simulink model "Robot"  (R2018a)
settings: Solver=VariableStepAuto  StartTime=0.0  StopTime=inf  FixedStep=1e-4  RelTol=1e-3  EnableMultiTasking=on
values from neighbouring files (symbols this model uses):
  CM730_acc_center = (4 * 9.80665)    (= 39.2266)    [CM730.m]
  CM730_acc_gain = 512 / CM730_acc_center    (= 13.0523675261)    [CM730.m]
  CM730_gyro_center = (1600 / 360 * 2 * pi)    (= 27.9252680319)    [CM730.m]
  CM730_gyro_gain = 512 / CM730_gyro_center    (= 18.3346494442)    [CM730.m]
  CM730_sample_time = 1e-3    (= 0.001)    [CM730.m]
  FSR_max = 254    [FSR.m]
  FSR_no_load = 255    [FSR.m]
  FSR_sample_time = 0.001    [FSR.m]
  FSR_scale = 1000    [FSR.m]
  g = 0    [Euler.m]
  MX106_Te = 1/1000    (= 0.001)    [MX106_init.m]
  MX28_inertia = 9e-8 * MX28_reduction^2    (= 0.0033385284)    [MX28_init.m]
  MX28_Te = 1/1000    (= 0.001)    [MX28_init.m]
  posZero_ID1 = posZero(1)    [Robot_init.m]
  posZero_ID10 = posZero(14)    [Robot_init.m]
  posZero_ID11 = posZero(9)    [Robot_init.m]
  posZero_ID12 = posZero(15)    [Robot_init.m]
  posZero_ID13 = posZero(10)    [Robot_init.m]
  posZero_ID14 = posZero(16)    [Robot_init.m]
  posZero_ID15 = posZero(11)    [Robot_init.m]
  posZero_ID16 = posZero(17)    [Robot_init.m]
  posZero_ID17 = posZero(12)    [Robot_init.m]
  posZero_ID18 = posZero(18)    [Robot_init.m]
  posZero_ID19 = posZero(19)    [Robot_init.m]
  posZero_ID2 = posZero(4)    [Robot_init.m]
  posZero_ID20 = posZero(20)    [Robot_init.m]
  posZero_ID3 = posZero(2)    [Robot_init.m]
  posZero_ID4 = posZero(5)    [Robot_init.m]
  posZero_ID5 = posZero(3)    [Robot_init.m]
  posZero_ID6 = posZero(6)    [Robot_init.m]
  posZero_ID7 = posZero(7)    [Robot_init.m]
  posZero_ID8 = posZero(13)    [Robot_init.m]
  posZero_ID9 = posZero(8)    [Robot_init.m]
  robot_chest_mass = 2385.0    (= 2385)    [Robot_init.m]
  robot_floor_friction_coeff = 0.6    [Robot_init.m]
  robot_floor_position_gain = -1e5    (= -100000)    [Robot_init.m]
  robot_floor_speed_gain = -1e3    (= -1000)    [Robot_init.m]
  robot_gravity = [0 0 0]    [Robot_init.m]
  robot_head_mass = 177.69    [Robot_init.m]
  robot_hip1_mass = 49.00    (= 49)    [Robot_init.m]
  robot_left_ankle_mass = 360.00    (= 360)    [Robot_init.m]
  robot_left_foot_mass = 267.00    (= 267)    [Robot_init.m]
  robot_left_forearm_mass = 248.00    (= 248)    [Robot_init.m]
  robot_left_hip2_mass = 358.00    (= 358)    [Robot_init.m]
  robot_left_lower_leg_mass = 129.00    (= 129)    [Robot_init.m]
  robot_left_shoulder_mass = 39.00    (= 39)    [Robot_init.m]
  robot_left_thigh_mass = 1263.00    (= 1263)    [Robot_init.m]
  robot_left_upper_arm_mass = 247.00    (= 247)    [Robot_init.m]
  robot_neck_mass = 90    [Robot_init.m]
  robot_right_ankle_mass = 360.00    (= 360)    [Robot_init.m]
  robot_right_foot_mass = 267.00    (= 267)    [Robot_init.m]
  robot_right_forearm_mass = 248.00    (= 248)    [Robot_init.m]
  robot_right_hip2_mass = 358.00    (= 358)    [Robot_init.m]
  robot_right_lower_leg_mass = 129.00    (= 129)    [Robot_init.m]
  robot_right_shoulder_mass = 39.00    (= 39)    [Robot_init.m]
  robot_right_thigh_mass = 263.00    (= 263)    [Robot_init.m]
  robot_right_upper_arm_mass = 247.00    (= 247)    [Robot_init.m]
  X = get(hObject,'Value')    [gui_kine.m]
  Y = get(hObject,'Value')    [gui_kine.m]
  Z = get(hObject,'Value')    [gui_kine.m]
libraries: sm_lib x167, fl_lib x128, nesl_utility x77, dspindex x1
(part 2 of 7)

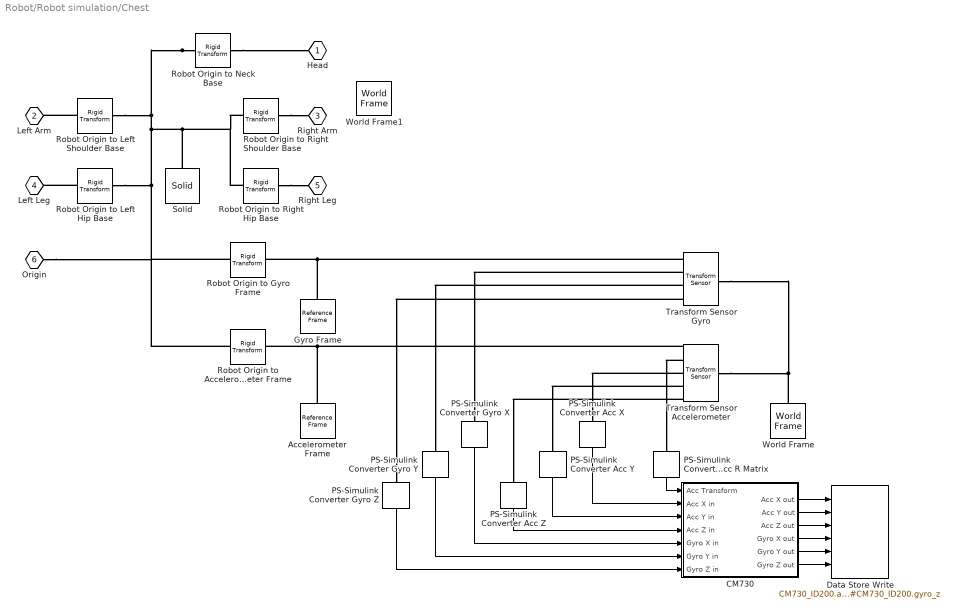
== system Robot/Robot simulation/Chest ==
  Accelerometer Frame : sm_lib/Frames and Transforms/Reference Frame
  CM730 : Subsystem  TreatAsAtomicUnit=on  SystemSampleTime=CM730_sample_time
  Data Store Write : DataStoreWrite  DataStoreName=CM730_ID200  DataStoreElements=CM730_ID200.acc_x#CM730_ID200.acc_y#CM730_ID200.acc_z#CM730_ID200.gyro_x#CM730_ID200.gyro_y#CM730_ID200.gyro_z
  Gyro Frame : sm_lib/Frames and Transforms/Reference Frame
  PS-Simulink Converter Acc R Matrix : nesl_utility/PS-Simulink Converter  PhysicalDomain=network_engine_domain  SubClassName=ps_output  LeftPortType=input  RightPortType=output  PseudoPeriodic=off  Frequencies=[]  Unit=1  AffineConversion=off
  PS-Simulink Converter Acc X : nesl_utility/PS-Simulink Converter  PhysicalDomain=network_engine_domain  SubClassName=ps_output  LeftPortType=input  RightPortType=output  PseudoPeriodic=off  Frequencies=[]  Unit=m/s^2  AffineConversion=off
  PS-Simulink Converter Acc Y : nesl_utility/PS-Simulink Converter  PhysicalDomain=network_engine_domain  SubClassName=ps_output  LeftPortType=input  RightPortType=output  PseudoPeriodic=off  Frequencies=[]  Unit=m/s^2  AffineConversion=off
  PS-Simulink Converter Acc Z : nesl_utility/PS-Simulink Converter  PhysicalDomain=network_engine_domain  SubClassName=ps_output  LeftPortType=input  RightPortType=output  PseudoPeriodic=off  Frequencies=[]  Unit=m/s^2  AffineConversion=off
  PS-Simulink Converter Gyro X : nesl_utility/PS-Simulink Converter  PhysicalDomain=network_engine_domain  SubClassName=ps_output  LeftPortType=input  RightPortType=output  PseudoPeriodic=off  Frequencies=[]  Unit=rad/s  AffineConversion=off
  PS-Simulink Converter Gyro Y : nesl_utility/PS-Simulink Converter  PhysicalDomain=network_engine_domain  SubClassName=ps_output  LeftPortType=input  RightPortType=output  PseudoPeriodic=off  Frequencies=[]  Unit=rad/s  AffineConversion=off
  PS-Simulink Converter Gyro Z : nesl_utility/PS-Simulink Converter  PhysicalDomain=network_engine_domain  SubClassName=ps_output  LeftPortType=input  RightPortType=output  PseudoPeriodic=off  Frequencies=[]  Unit=rad/s  AffineConversion=off
  Robot Origin to Accelerometer Frame : sm_lib/Frames and Transforms/Rigid Transform  TranslationMethod=Cartesian  TranslationStandardOffset=0  TranslationLengthUnit=mm  TranslationStandardAxis=+Z  TranslationCartesianOffset=robot_origin_to_acc_tra  TranslationROffset=0  TranslationROffsetUnits=m  TranslationZOffset=0  TranslationZOffsetUnits=m  TranslationThetaOffset=0  TranslationThetaOffsetUnits=deg  RotationMethod=RotationMatrix  RotationAngleUnits=deg  RotationStandardAxis=+Z  RotationAngle=0  RotationArbitraryAxis=[0 0 1]  FollAlignAxisA=+X  BaseAlignAxisA=-Y  FollAlignAxisB=+Z  BaseAlignAxisB=+Z  RotationSequenceAxes=FollowerAxes  RotationSequence=XYX  RotationSequenceAngles=[0 0 0]  RotationSequenceAnglesUnits=deg  RotationMatrix=robot_origin_to_acc_rot
  Robot Origin to Gyro Frame : sm_lib/Frames and Transforms/Rigid Transform  TranslationMethod=Cartesian  TranslationStandardOffset=0  TranslationLengthUnit=mm  TranslationStandardAxis=+Z  TranslationCartesianOffset=robot_origin_to_gyro_tra  TranslationROffset=0  TranslationROffsetUnits=m  TranslationZOffset=0  TranslationZOffsetUnits=m  TranslationThetaOffset=0  TranslationThetaOffsetUnits=deg  RotationMethod=RotationMatrix  RotationAngleUnits=deg  RotationStandardAxis=+Z  RotationAngle=0  RotationArbitraryAxis=[0 0 1]  FollAlignAxisA=+X  BaseAlignAxisA=-Y  FollAlignAxisB=+Z  BaseAlignAxisB=-Z  RotationSequenceAxes=FollowerAxes  RotationSequence=XYX  RotationSequenceAngles=[0 0 0]  RotationSequenceAnglesUnits=deg  RotationMatrix=robot_origin_to_gyro_rot
  Robot Origin to Left Hip Base : sm_lib/Frames and Transforms/Rigid Transform  TranslationMethod=Cartesian  TranslationStandardOffset=0  TranslationLengthUnit=mm  TranslationStandardAxis=+Z  TranslationCartesianOffset=robot_origin_to_left_hip_base_tra  TranslationROffset=0  TranslationROffsetUnits=m  TranslationZOffset=0  TranslationZOffsetUnits=m  TranslationThetaOffset=0  TranslationThetaOffsetUnits=deg  RotationMethod=RotationMatrix  RotationAngleUnits=deg  RotationStandardAxis=+Z  RotationAngle=0  RotationArbitraryAxis=[0 0 1]  FollAlignAxisA=+X  BaseAlignAxisA=-Y  FollAlignAxisB=+Y  BaseAlignAxisB=-X  RotationSequenceAxes=FollowerAxes  RotationSequence=XYX  RotationSequenceAngles=[0 0 0]  RotationSequenceAnglesUnits=deg  RotationMatrix=robot_origin_to_left_hip_base_rot
  Robot Origin to Left Shoulder Base : sm_lib/Frames and Transforms/Rigid Transform  TranslationMethod=Cartesian  TranslationStandardOffset=0  TranslationLengthUnit=mm  TranslationStandardAxis=+Z  TranslationCartesianOffset=robot_origin_to_left_shoulder_base_tra  TranslationROffset=0  TranslationROffsetUnits=m  TranslationZOffset=0  TranslationZOffsetUnits=m  TranslationThetaOffset=0  TranslationThetaOffsetUnits=deg  RotationMethod=RotationMatrix  RotationAngleUnits=deg  RotationStandardAxis=+Z  RotationAngle=0  RotationArbitraryAxis=[0 0 1]  FollAlignAxisA=+X  BaseAlignAxisA=+Y  FollAlignAxisB=+Y  BaseAlignAxisB=+Z  RotationSequenceAxes=FollowerAxes  RotationSequence=XYX  RotationSequenceAngles=[0 0 0]  RotationSequenceAnglesUnits=deg  RotationMatrix=robot_origin_to_left_shoulder_base_rot
  Robot Origin to Neck Base : sm_lib/Frames and Transforms/Rigid Transform  TranslationMethod=Cartesian  TranslationStandardOffset=0  TranslationLengthUnit=mm  TranslationStandardAxis=+Z  TranslationCartesianOffset=robot_origin_to_neck_base_tra  TranslationROffset=0  TranslationROffsetUnits=m  TranslationZOffset=0  TranslationZOffsetUnits=m  TranslationThetaOffset=0  TranslationThetaOffsetUnits=deg  RotationMethod=RotationMatrix  RotationAngleUnits=deg  RotationStandardAxis=+Z  RotationAngle=0  RotationArbitraryAxis=[0 0 1]  FollAlignAxisA=+X  BaseAlignAxisA=+Y  FollAlignAxisB=+Y  BaseAlignAxisB=+Z  RotationSequenceAxes=FollowerAxes  RotationSequence=XYX  RotationSequenceAngles=[0 0 0]  RotationSequenceAnglesUnits=deg  RotationMatrix=robot_origin_to_neck_base_rot
  Robot Origin to Right Hip Base : sm_lib/Frames and Transforms/Rigid Transform  TranslationMethod=Cartesian  TranslationStandardOffset=0  TranslationLengthUnit=mm  TranslationStandardAxis=+Z  TranslationCartesianOffset=robot_origin_to_right_hip_base_tra  TranslationROffset=0  TranslationROffsetUnits=m  TranslationZOffset=0  TranslationZOffsetUnits=m  TranslationThetaOffset=0  TranslationThetaOffsetUnits=deg  RotationMethod=RotationMatrix  RotationAngleUnits=deg  RotationStandardAxis=+Z  RotationAngle=0  RotationArbitraryAxis=[0 0 1]  FollAlignAxisA=+X  BaseAlignAxisA=-Y  FollAlignAxisB=+Y  BaseAlignAxisB=-X  RotationSequenceAxes=FollowerAxes  RotationSequence=XYX  RotationSequenceAngles=[0 0 0]  RotationSequenceAnglesUnits=deg  RotationMatrix=robot_origin_to_right_hip_base_rot
  Robot Origin to Right Shoulder Base : sm_lib/Frames and Transforms/Rigid Transform  TranslationMethod=Cartesian  TranslationStandardOffset=0  TranslationLengthUnit=mm  TranslationStandardAxis=+Z  TranslationCartesianOffset=robot_origin_to_right_shoulder_base_tra  TranslationROffset=0  TranslationROffsetUnits=m  TranslationZOffset=0  TranslationZOffsetUnits=m  TranslationThetaOffset=0  TranslationThetaOffsetUnits=deg  RotationMethod=RotationMatrix  RotationAngleUnits=deg  RotationStandardAxis=+Z  RotationAngle=0  RotationArbitraryAxis=[0 0 1]  FollAlignAxisA=-Z  BaseAlignAxisA=+X  FollAlignAxisB=-X  BaseAlignAxisB=+Y  RotationSequenceAxes=FollowerAxes  RotationSequence=XYX  RotationSequenceAngles=[0 0 0]  RotationSequenceAnglesUnits=deg  RotationMatrix=robot_origin_to_right_shoulder_base_rot
  Solid : sm_lib/Body Elements/Solid  InertiaType=Custom  Mass=robot_chest_mass  MassUnits=g  CenterOfMass=robot_origin_to_center_mass  CenterOfMassUnits=mm  MomentsOfInertia=robot_chest_moment_inertia  MomentsOfInertiaUnits=g*mm^2  ProductsOfInertia=robot_chest_product_inertia  ProductsOfInertiaUnits=g*mm^2  DensityBased=on  Density=1000  DensityUnits=kg/(m^3)  DoExposeReferenceFrame=on  SerializedFrames=<Frames/>  GraphicType=FromGeometry  MarkerShape=Sphere  MarkerSize=10  MarkerSizeUnits=m  GraphicVisPropType=SimpleVisualProperties  GraphicDiffuseColor=[0.5 0.5 0.5]  GraphicSpecularColor=[0.5 0.5 0.5 1.0]  GraphicAmbientColor=[0.15 0.15 0.15 1.0]  GraphicEmissiveColor=[0.0 0.0 0.0 1.0]  GraphicShininess=75  GraphicOpacity=1.0  GeometryShape=FromFile  RectangleSize=[1 1]  RectangleSizeUnits=m  BrickDimensions=[115.5 112.1 47.8]  BrickDimensionUnits=mm  CylinderRadius=1  CylinderRadiusUnits=m  CylinderLength=1  CylinderLengthUnits=m  SphereRadius=1  SphereRadiusUnits=m  EllipsoidRadii=[1 1 1]  EllipsoidRadiiUnits=m  ExtrusionCrossSection=[1 1; -1 1; -1 -1; 1 -1]  ExtrusionCrossSectionUnits=m  ExtrusionLength=1  ExtrusionLengthUnits=m  PolygonNumSides=3  PolygonOuterRadius=1  PolygonOuterRadiusUnits=m  ExtGeomFileType=STL  ExtGeomFileName=\STL\Chest.STL  ExtGeomFileUnits=mm  RevolutionCrossSection=[1 1; 1 -1; 2 -1; 2 1]  RevolutionCrossSectionUnits=m  RevolutionExtent=Full  RevolutionAngle=180  RevolutionAngleUnits=deg
  Transform Sensor Accelerometer : sm_lib/Frames and Transforms/Transform Sensor  MeasurementFrame=Follower  SenseAngle=off  SenseAxis=off  SenseAngle1=off  SenseAngle2=off  SenseAngle3=off  SenseQ=off  SenseR=on  SenseOmegaX=off  SenseOmegaY=off  SenseOmegaZ=off  SenseOmega1=off  SenseOmega2=off  SenseOmega3=off  SenseQDot=off  SenseRDot=off  SenseAlphaX=off  SenseAlphaY=off  SenseAlphaZ=off  SenseAlpha1=off  SenseAlpha2=off  SenseAlpha3=off  SenseQDDot=off  SenseRDDot=off  SenseX=off  SenseY=off  SenseZ=off  SenseRad=off  SenseAzim=off  SenseDist=off  SenseInc=off  SenseXDot=off  SenseYDot=off  SenseZDot=off  SenseRadDot=off  SenseAzimDot=off  SenseDistDot=off  SenseIncDot=off  SenseXDDot=on  SenseYDDot=on  SenseZDDot=on  SenseRadDDot=off  SenseAzimDDot=off  SenseDistDDot=off  SenseIncDDot=off
  Transform Sensor Gyro : sm_lib/Frames and Transforms/Transform Sensor  MeasurementFrame=Follower  SenseAngle=off  SenseAxis=off  SenseAngle1=off  SenseAngle2=off  SenseAngle3=off  SenseQ=off  SenseR=off  SenseOmegaX=on  SenseOmegaY=on  SenseOmegaZ=on  SenseOmega1=off  SenseOmega2=off  SenseOmega3=off  SenseQDot=off  SenseRDot=off  SenseAlphaX=off  SenseAlphaY=off  SenseAlphaZ=off  SenseAlpha1=off  SenseAlpha2=off  SenseAlpha3=off  SenseQDDot=off  SenseRDDot=off  SenseX=off  SenseY=off  SenseZ=off  SenseRad=off  SenseAzim=off  SenseDist=off  SenseInc=off  SenseXDot=off  SenseYDot=off  SenseZDot=off  SenseRadDot=off  SenseAzimDot=off  SenseDistDot=off  SenseIncDot=off  SenseXDDot=off  SenseYDDot=off  SenseZDDot=off  SenseRadDDot=off  SenseAzimDDot=off  SenseDistDDot=off  SenseIncDDot=off
  World Frame : sm_lib/Frames and Transforms/World Frame
  World Frame1 : sm_lib/Frames and Transforms/World Frame
  Head : PMIOPort  Side=Right
  Left Arm : PMIOPort  Port=2  Side=Left
  Right Arm : PMIOPort  Port=3  Side=Right
  Left Leg : PMIOPort  Port=4  Side=Left
  Right Leg : PMIOPort  Port=5  Side=Right
  Origin : PMIOPort  Port=6  Side=Left
  wires:
  CM730/1(Acc X out) -> Data Store Write/1
  CM730/2(Acc Y out) -> Data Store Write/2
  CM730/3(Acc Z out) -> Data Store Write/3
  CM730/4(Gyro X out) -> Data Store Write/4
  CM730/5(Gyro Y out) -> Data Store Write/5
  CM730/6(Gyro Z out) -> Data Store Write/6
  PS-Simulink Converter Acc X/1 -> CM730/2(Acc X in)
  PS-Simulink Converter Acc Y/1 -> CM730/3(Acc Y in)
  PS-Simulink Converter Acc Z/1 -> CM730/4(Acc Z in)
  PS-Simulink Converter Gyro X/1 -> CM730/5(Gyro X in)
  PS-Simulink Converter Gyro Z/1 -> CM730/7(Gyro Z in)
  PS-Simulink Converter Gyro Y/1 -> CM730/6(Gyro Y in)
  PS-Simulink Converter Acc R Matrix/1 -> CM730/1(Acc Transform)
  connections:
  Robot Origin to Neck Base/RConn1 -- Head/RConn1
  Robot Origin to Right Shoulder Base/RConn1 -- Right Arm/RConn1
  Robot Origin to Right Hip Base/RConn1 -- Right Leg/RConn1
  Robot Origin to Neck Base/LConn1 -- Robot Origin to Left Shoulder Base/LConn1 -- Robot Origin to Accelerometer Frame/LConn1 -- Origin/RConn1 -- Robot Origin to Gyro Frame/LConn1 -- Robot Origin to Left Hip Base/LConn1 -- Robot Origin to Right Hip Base/LConn1 -- Robot Origin to Right Shoulder Base/LConn1 -- Solid/RConn1
  Robot Origin to Left Shoulder Base/RConn1 -- Left Arm/RConn1
  Robot Origin to Left Hip Base/RConn1 -- Left Leg/RConn1
  Gyro Frame/RConn1 -- Transform Sensor Gyro/RConn1 -- Robot Origin to Gyro Frame/RConn1
  Accelerometer Frame/RConn1 -- Transform Sensor Accelerometer/RConn1 -- Robot Origin to Accelerometer Frame/RConn1
  World Frame/RConn1 -- Transform Sensor Gyro/LConn1 -- Transform Sensor Accelerometer/LConn1
  Transform Sensor Gyro/RConn2 -- PS-Simulink Converter Gyro X/LConn1
  Transform Sensor Gyro/RConn3 -- PS-Simulink Converter Gyro Y/LConn1
  Transform Sensor Gyro/RConn4 -- PS-Simulink Converter Gyro Z/LConn1
  Transform Sensor Accelerometer/RConn2 -- PS-Simulink Converter Acc R Matrix/LConn1
  Transform Sensor Accelerometer/RConn5 -- PS-Simulink Converter Acc Z/LConn1
  Transform Sensor Accelerometer/RConn4 -- PS-Simulink Converter Acc Y/LConn1
  Transform Sensor Accelerometer/RConn3 -- PS-Simulink Converter Acc X/LConn1

== system Robot/Robot simulation/Head ==
  Camera Endefector : sm_lib/Frames and Transforms/Reference Frame
  Head : Subsystem
  Head Axis : sm_lib/Frames and Transforms/Reference Frame
  Head Origin : sm_lib/Frames and Transforms/Reference Frame
  Head Pan (19) : Subsystem
  Head Tilt (20) : Subsystem
  Neck : Subsystem
  Neck Axis : sm_lib/Frames and Transforms/Reference Frame
  Neck Base : sm_lib/Frames and Transforms/Reference Frame
  Chest : PMIOPort  Side=Left
  connections:
  Neck Axis/RConn1 -- Head Pan (19)/RConn1 -- Neck/LConn1
  Neck Base/RConn1 -- Head Pan (19)/LConn1 -- Chest/RConn1
  Head Tilt (20)/RConn1 -- Head Axis/RConn1 -- Head/LConn1
  Neck/RConn1 -- Head Tilt (20)/LConn1 -- Head Origin/RConn1
  Head/RConn1 -- Camera Endefector/RConn1

== system Robot/Robot simulation/Left Arm ==
  Left Arm Axis : sm_lib/Frames and Transforms/Reference Frame
  Left Arm Base : sm_lib/Frames and Transforms/Reference Frame
  Left Elbow (6) : Subsystem
  Left Endefector : sm_lib/Frames and Transforms/Reference Frame
  Left Forearm : Subsystem
  Left Forearm Axis : sm_lib/Frames and Transforms/Reference Frame
  Left Forearm Base : sm_lib/Frames and Transforms/Reference Frame
  Left Shoulder : Subsystem
  Left Shoulder Axis : sm_lib/Frames and Transforms/Reference Frame
  Left Shoulder Base : sm_lib/Frames and Transforms/Reference Frame
  Left Shoulder Pitch (2) : Subsystem
  Left Shoulder Roll (4) : Subsystem
  Left Upper Arm : Subsystem
  Chest : PMIOPort  Side=Right
  connections:
  Chest/RConn1 -- Left Shoulder Pitch (2)/LConn1 -- Left Shoulder Base/RConn1
  Left Shoulder Axis/RConn1 -- Left Shoulder Pitch (2)/RConn1 -- Left Shoulder/LConn1
  Left Upper Arm/RConn1 -- Left Elbow (6)/LConn1 -- Left Forearm Base/RConn1
  Left Forearm Axis/RConn1 -- Left Elbow (6)/RConn1 -- Left Forearm/LConn1
  Left Shoulder/RConn1 -- Left Shoulder Roll (4)/LConn1 -- Left Arm Axis/RConn1
  Left Upper Arm/LConn1 -- Left Shoulder Roll (4)/RConn1 -- Left Arm Base/RConn1
  Left Forearm/RConn1 -- Left Endefector/RConn1

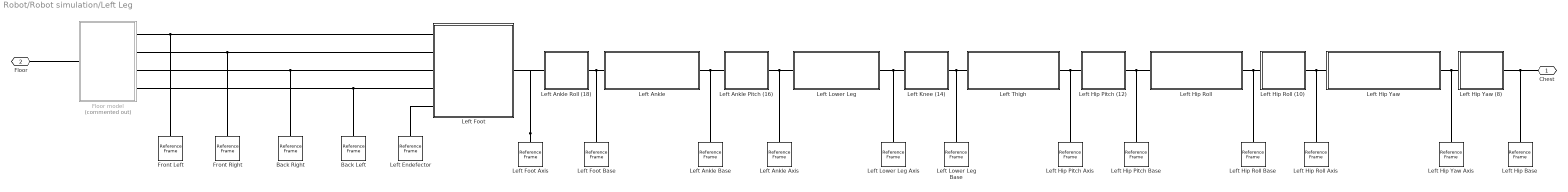
== system Robot/Robot simulation/Left Leg ==
  Back Left : sm_lib/Frames and Transforms/Reference Frame
  Back Right : sm_lib/Frames and Transforms/Reference Frame
  Floor model : Subsystem  Commented=on
  Front Left : sm_lib/Frames and Transforms/Reference Frame
  Front Right : sm_lib/Frames and Transforms/Reference Frame
  Left Ankle : Subsystem
  Left Ankle Axis : sm_lib/Frames and Transforms/Reference Frame
  Left Ankle Base : sm_lib/Frames and Transforms/Reference Frame
  Left Ankle Pitch (16) : Subsystem
  Left Ankle Roll (18) : Subsystem
  Left Endefector : sm_lib/Frames and Transforms/Reference Frame
  Left Foot : Subsystem
  Left Foot Axis : sm_lib/Frames and Transforms/Reference Frame
  Left Foot Base : sm_lib/Frames and Transforms/Reference Frame
  Left Hip Base : sm_lib/Frames and Transforms/Reference Frame
  Left Hip Pitch (12) : Subsystem
  Left Hip Pitch Axis : sm_lib/Frames and Transforms/Reference Frame
  Left Hip Pitch Base : sm_lib/Frames and Transforms/Reference Frame
  Left Hip Roll : Subsystem
  Left Hip Roll (10) : Subsystem
  Left Hip Roll Axis : sm_lib/Frames and Transforms/Reference Frame
  Left Hip Roll Base : sm_lib/Frames and Transforms/Reference Frame
  Left Hip Yaw : Subsystem
  Left Hip Yaw (8) : Subsystem
  Left Hip Yaw Axis : sm_lib/Frames and Transforms/Reference Frame
  Left Knee (14) : Subsystem
  Left Lower Leg : Subsystem
  Left Lower Leg Axis : sm_lib/Frames and Transforms/Reference Frame
  Left Lower Leg Base : sm_lib/Frames and Transforms/Reference Frame
  Left Thigh : Subsystem
  Chest : PMIOPort  Side=Right
  Floor : PMIOPort  Port=2  Side=Left
  connections:
  Chest/RConn1 -- Left Hip Yaw (8)/LConn1 -- Left Hip Base/RConn1
  Left Hip Roll/RConn1 -- Left Hip Pitch (12)/LConn1 -- Left Hip Pitch Base/RConn1
  Left Thigh/RConn1 -- Left Knee (14)/LConn1 -- Left Lower Leg Base/RConn1
  Left Lower Leg/RConn1 -- Left Ankle Pitch (16)/RConn1 -- Left Ankle Axis/RConn1
  Left Ankle/RConn1 -- Left Ankle Roll (18)/LConn1 -- Left Foot Base/RConn1
  Left Hip Yaw/LConn1 -- Left Hip Yaw (8)/RConn1 -- Left Hip Yaw Axis/RConn1
  Left Hip Roll Axis/RConn1 -- Left Hip Roll (10)/RConn1 -- Left Hip Yaw/RConn1
  Left Hip Roll Base/RConn1 -- Left Hip Roll (10)/LConn1 -- Left Hip Roll/LConn1
  Left Thigh/LConn1 -- Left Hip Pitch (12)/RConn1 -- Left Hip Pitch Axis/RConn1
  Left Lower Leg/LConn1 -- Left Knee (14)/RConn1 -- Left Lower Leg Axis/RConn1
  Left Ankle/LConn1 -- Left Ankle Pitch (16)/LConn1 -- Left Ankle Base/RConn1
  Left Foot Axis/RConn1 -- Left Foot/LConn1 -- Left Ankle Roll (18)/RConn1
  Left Foot/RConn1 -- Front Left/RConn1 -- Floor model/LConn1
  Front Right/RConn1 -- Floor model/LConn2 -- Left Foot/RConn2
  Back Right/RConn1 -- Floor model/LConn3 -- Left Foot/RConn3
  Back Left/RConn1 -- Floor model/LConn4 -- Left Foot/RConn4
  Floor/RConn1 -- Floor model/RConn1
  Left Foot/RConn5 -- Left Endefector/RConn1

== system Robot/Robot simulation/Right Arm ==
  Right Arm Axis : sm_lib/Frames and Transforms/Reference Frame
  Right Arm Base : sm_lib/Frames and Transforms/Reference Frame
  Right Elbow (5) : Subsystem
  Right Endefector : sm_lib/Frames and Transforms/Reference Frame
  Right ForeArm Axis : sm_lib/Frames and Transforms/Reference Frame
  Right ForeArm Base : sm_lib/Frames and Transforms/Reference Frame
  Right Forearm : Subsystem
  Right Shoulder : Subsystem
  Right Shoulder Axis : sm_lib/Frames and Transforms/Reference Frame
  Right Shoulder Base : sm_lib/Frames and Transforms/Reference Frame
  Right Shoulder Pitch (1) : Subsystem
  Right Shoulder Roll (3) : Subsystem
  Right Upper Arm : Subsystem
  Chest : PMIOPort  Side=Left
  connections:
  Chest/RConn1 -- Right Shoulder Pitch (1)/LConn1 -- Right Shoulder Base/RConn1
  Right Shoulder Axis/RConn1 -- Right Shoulder Pitch (1)/RConn1 -- Right Shoulder/LConn1
  Right Upper Arm/RConn1 -- Right Elbow (5)/LConn1 -- Right ForeArm Base/RConn1
  Right ForeArm Axis/RConn1 -- Right Elbow (5)/RConn1 -- Right Forearm/LConn1
  Right Shoulder/RConn1 -- Right Shoulder Roll (3)/LConn1 -- Right Arm Axis/RConn1
  Right Upper Arm/LConn1 -- Right Shoulder Roll (3)/RConn1 -- Right Arm Base/RConn1
  Right Endefector/RConn1 -- Right Forearm/RConn1

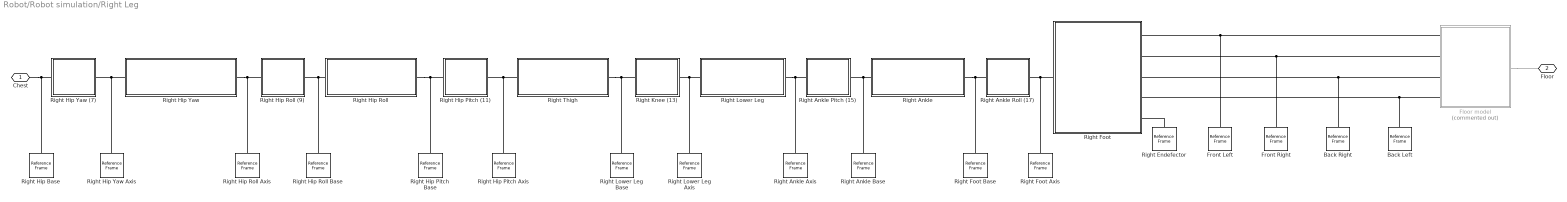
== system Robot/Robot simulation/Right Leg ==
  Back Left : sm_lib/Frames and Transforms/Reference Frame
  Back Right : sm_lib/Frames and Transforms/Reference Frame
  Floor model : Subsystem  Commented=on
  Front Left : sm_lib/Frames and Transforms/Reference Frame
  Front Right : sm_lib/Frames and Transforms/Reference Frame
  Right Ankle : Subsystem
  Right Ankle Axis : sm_lib/Frames and Transforms/Reference Frame
  Right Ankle Base : sm_lib/Frames and Transforms/Reference Frame
  Right Ankle Pitch (15) : Subsystem
  Right Ankle Roll (17) : Subsystem
  Right Endefector : sm_lib/Frames and Transforms/Reference Frame
  Right Foot : Subsystem
  Right Foot Axis : sm_lib/Frames and Transforms/Reference Frame
  Right Foot Base : sm_lib/Frames and Transforms/Reference Frame
  Right Hip Base : sm_lib/Frames and Transforms/Reference Frame
  Right Hip Pitch (11) : Subsystem
  Right Hip Pitch Axis : sm_lib/Frames and Transforms/Reference Frame
  Right Hip Pitch Base : sm_lib/Frames and Transforms/Reference Frame
  Right Hip Roll : Subsystem
  Right Hip Roll (9) : Subsystem
  Right Hip Roll Axis : sm_lib/Frames and Transforms/Reference Frame
  Right Hip Roll Base : sm_lib/Frames and Transforms/Reference Frame
  Right Hip Yaw : Subsystem
  Right Hip Yaw (7) : Subsystem
  Right Hip Yaw Axis : sm_lib/Frames and Transforms/Reference Frame
  Right Knee (13) : Subsystem
  Right Lower Leg : Subsystem
  Right Lower Leg Axis : sm_lib/Frames and Transforms/Reference Frame
  Right Lower Leg Base : sm_lib/Frames and Transforms/Reference Frame
  Right Thigh : Subsystem
  Chest : PMIOPort  Side=Left
  Floor : PMIOPort  Port=2  Side=Right
  connections:
  Chest/RConn1 -- Right Hip Yaw (7)/LConn1 -- Right Hip Base/RConn1
  Right Hip Yaw Axis/RConn1 -- Right Hip Yaw (7)/RConn1 -- Right Hip Yaw/LConn1
  Right Hip Yaw/RConn1 -- Right Hip Roll (9)/RConn1 -- Right Hip Roll Axis/RConn1
  Right Hip Roll/RConn1 -- Right Hip Pitch (11)/LConn1 -- Right Hip Pitch Base/RConn1
  Right Thigh/RConn1 -- Right Knee (13)/LConn1 -- Right Lower Leg Base/RConn1
  Right Ankle/RConn1 -- Right Ankle Roll (17)/LConn1 -- Right Foot Base/RConn1
  Right Hip Roll/LConn1 -- Right Hip Roll (9)/LConn1 -- Right Hip Roll Base/RConn1
  Right Thigh/LConn1 -- Right Hip Pitch (11)/RConn1 -- Right Hip Pitch Axis/RConn1
  Right Lower Leg/LConn1 -- Right Knee (13)/RConn1 -- Right Lower Leg Axis/RConn1
  Right Lower Leg/RConn1 -- Right Ankle Axis/RConn1 -- Right Ankle Pitch (15)/RConn1
  Right Ankle/LConn1 -- Right Ankle Pitch (15)/LConn1 -- Right Ankle Base/RConn1
  Right Foot/LConn1 -- Right Foot Axis/RConn1 -- Right Ankle Roll (17)/RConn1
  Front Left/RConn1 -- Floor model/LConn1 -- Right Foot/RConn1
  Front Right/RConn1 -- Floor model/LConn2 -- Right Foot/RConn2
  Back Right/RConn1 -- Floor model/LConn3 -- Right Foot/RConn3
  Back Left/RConn1 -- Floor model/LConn4 -- Right Foot/RConn4
  Floor model/RConn1 -- Floor/RConn1
  Right Endefector/RConn1 -- Right Foot/RConn5

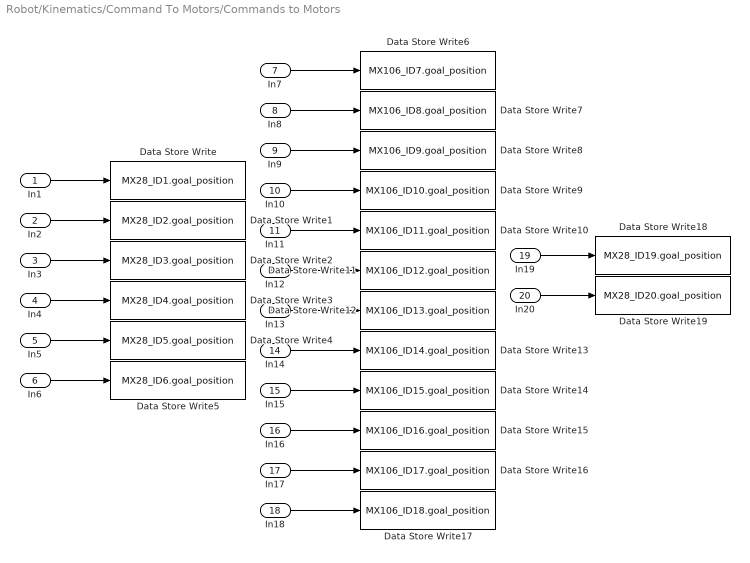
== system Robot/Kinematics/Command To Motors/Commands to Motors ==
  In1 : Inport
  In2 : Inport  Port=2
  In3 : Inport  Port=3
  In4 : Inport  Port=4
  In5 : Inport  Port=5
  In6 : Inport  Port=6
  In7 : Inport  Port=7
  In8 : Inport  Port=8
  In9 : Inport  Port=9
  In10 : Inport  Port=10
  In11 : Inport  Port=11
  In12 : Inport  Port=12
  In13 : Inport  Port=13
  In14 : Inport  Port=14
  In15 : Inport  Port=15
  In16 : Inport  Port=16
  In17 : Inport  Port=17
  In18 : Inport  Port=18
  In19 : Inport  Port=19
  In20 : Inport  Port=20
  Data Store Write : DataStoreWrite  DataStoreName=MX28_ID1  DataStoreElements=MX28_ID1.goal_position
  Data Store Write1 : DataStoreWrite  DataStoreName=MX28_ID2  DataStoreElements=MX28_ID2.goal_position
  Data Store Write10 : DataStoreWrite  DataStoreName=MX106_ID11  DataStoreElements=MX106_ID11.goal_position
  Data Store Write11 : DataStoreWrite  DataStoreName=MX106_ID12  DataStoreElements=MX106_ID12.goal_position
  Data Store Write12 : DataStoreWrite  DataStoreName=MX106_ID13  DataStoreElements=MX106_ID13.goal_position
  Data Store Write13 : DataStoreWrite  DataStoreName=MX106_ID14  DataStoreElements=MX106_ID14.goal_position
  Data Store Write14 : DataStoreWrite  DataStoreName=MX106_ID15  DataStoreElements=MX106_ID15.goal_position
  Data Store Write15 : DataStoreWrite  DataStoreName=MX106_ID16  DataStoreElements=MX106_ID16.goal_position
  Data Store Write16 : DataStoreWrite  DataStoreName=MX106_ID17  DataStoreElements=MX106_ID17.goal_position
  Data Store Write17 : DataStoreWrite  DataStoreName=MX106_ID18  DataStoreElements=MX106_ID18.goal_position
  Data Store Write18 : DataStoreWrite  DataStoreName=MX28_ID19  DataStoreElements=MX28_ID19.goal_position
  Data Store Write19 : DataStoreWrite  DataStoreName=MX28_ID20  DataStoreElements=MX28_ID20.goal_position
  Data Store Write2 : DataStoreWrite  DataStoreName=MX28_ID3  DataStoreElements=MX28_ID3.goal_position
  Data Store Write3 : DataStoreWrite  DataStoreName=MX28_ID4  DataStoreElements=MX28_ID4.goal_position
  Data Store Write4 : DataStoreWrite  DataStoreName=MX28_ID5  DataStoreElements=MX28_ID5.goal_position
  Data Store Write5 : DataStoreWrite  DataStoreName=MX28_ID6  DataStoreElements=MX28_ID6.goal_position
  Data Store Write6 : DataStoreWrite  DataStoreName=MX106_ID7  DataStoreElements=MX106_ID7.goal_position
  Data Store Write7 : DataStoreWrite  DataStoreName=MX106_ID8  DataStoreElements=MX106_ID8.goal_position
  Data Store Write8 : DataStoreWrite  DataStoreName=MX106_ID9  DataStoreElements=MX106_ID9.goal_position
  Data Store Write9 : DataStoreWrite  DataStoreName=MX106_ID10  DataStoreElements=MX106_ID10.goal_position
  wires:
  In15/1 -> Data Store Write14/1
  In4/1 -> Data Store Write3/1
  In14/1 -> Data Store Write13/1
  In11/1 -> Data Store Write10/1
  In17/1 -> Data Store Write16/1
  In18/1 -> Data Store Write17/1
  In10/1 -> Data Store Write9/1
  In5/1 -> Data Store Write4/1
  In13/1 -> Data Store Write12/1
  In8/1 -> Data Store Write7/1
  In16/1 -> Data Store Write15/1
  In7/1 -> Data Store Write6/1
  In3/1 -> Data Store Write2/1
  In19/1 -> Data Store Write18/1
  In9/1 -> Data Store Write8/1
  In6/1 -> Data Store Write5/1
  In20/1 -> Data Store Write19/1
  In1/1 -> Data Store Write/1
  In12/1 -> Data Store Write11/1
  In2/1 -> Data Store Write1/1

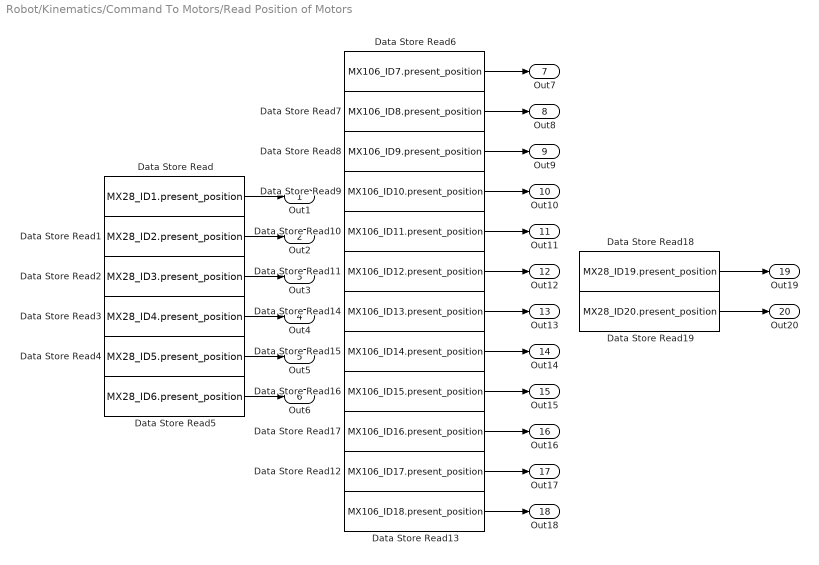
== system Robot/Kinematics/Command To Motors/Read Position of Motors ==
  Data Store Read : DataStoreRead  DataStoreName=MX28_ID1  DataStoreElements=MX28_ID1.present_position
  Data Store Read1 : DataStoreRead  DataStoreName=MX28_ID2  DataStoreElements=MX28_ID2.present_position
  Data Store Read10 : DataStoreRead  DataStoreName=MX106_ID11  DataStoreElements=MX106_ID11.present_position
  Data Store Read11 : DataStoreRead  DataStoreName=MX106_ID12  DataStoreElements=MX106_ID12.present_position
  Data Store Read12 : DataStoreRead  DataStoreName=MX106_ID17  DataStoreElements=MX106_ID17.present_position
  Data Store Read13 : DataStoreRead  DataStoreName=MX106_ID18  DataStoreElements=MX106_ID18.present_position
  Data Store Read14 : DataStoreRead  DataStoreName=MX106_ID13  DataStoreElements=MX106_ID13.present_position
  Data Store Read15 : DataStoreRead  DataStoreName=MX106_ID14  DataStoreElements=MX106_ID14.present_position
  Data Store Read16 : DataStoreRead  DataStoreName=MX106_ID15  DataStoreElements=MX106_ID15.present_position
  Data Store Read17 : DataStoreRead  DataStoreName=MX106_ID16  DataStoreElements=MX106_ID16.present_position
  Data Store Read18 : DataStoreRead  DataStoreName=MX28_ID19  DataStoreElements=MX28_ID19.present_position
  Data Store Read19 : DataStoreRead  DataStoreName=MX28_ID20  DataStoreElements=MX28_ID20.present_position
  Data Store Read2 : DataStoreRead  DataStoreName=MX28_ID3  DataStoreElements=MX28_ID3.present_position
  Data Store Read3 : DataStoreRead  DataStoreName=MX28_ID4  DataStoreElements=MX28_ID4.present_position
  Data Store Read4 : DataStoreRead  DataStoreName=MX28_ID5  DataStoreElements=MX28_ID5.present_position
  Data Store Read5 : DataStoreRead  DataStoreName=MX28_ID6  DataStoreElements=MX28_ID6.present_position
  Data Store Read6 : DataStoreRead  DataStoreName=MX106_ID7  DataStoreElements=MX106_ID7.present_position
  Data Store Read7 : DataStoreRead  DataStoreName=MX106_ID8  DataStoreElements=MX106_ID8.present_position
  Data Store Read8 : DataStoreRead  DataStoreName=MX106_ID9  DataStoreElements=MX106_ID9.present_position
  Data Store Read9 : DataStoreRead  DataStoreName=MX106_ID10  DataStoreElements=MX106_ID10.present_position
  Out1 : Outport
  Out2 : Outport  Port=2
  Out3 : Outport  Port=3
  Out4 : Outport  Port=4
  Out5 : Outport  Port=5
  Out6 : Outport  Port=6
  Out7 : Outport  Port=7
  Out8 : Outport  Port=8
  Out9 : Outport  Port=9
  Out10 : Outport  Port=10
  Out11 : Outport  Port=11
  Out12 : Outport  Port=12
  Out13 : Outport  Port=13
  Out14 : Outport  Port=14
  Out15 : Outport  Port=15
  Out16 : Outport  Port=16
  Out17 : Outport  Port=17
  Out18 : Outport  Port=18
  Out19 : Outport  Port=19
  Out20 : Outport  Port=20
  wires:
  Data Store Read12/1 -> Out17/1
  Data Store Read1/1 -> Out2/1
  Data Store Read18/1 -> Out19/1
  Data Store Read10/1 -> Out11/1
  Data Store Read6/1 -> Out7/1
  Data Store Read14/1 -> Out13/1
  Data Store Read3/1 -> Out4/1
  Data Store Read9/1 -> Out10/1
  Data Store Read7/1 -> Out8/1
  Data Store Read8/1 -> Out9/1
  Data Store Read13/1 -> Out18/1
  Data Store Read2/1 -> Out3/1
  Data Store Read4/1 -> Out5/1
  Data Store Read11/1 -> Out12/1
  Data Store Read/1 -> Out1/1
  Data Store Read5/1 -> Out6/1
  Data Store Read15/1 -> Out14/1
  Data Store Read16/1 -> Out15/1
  Data Store Read17/1 -> Out16/1
  Data Store Read19/1 -> Out20/1

== system Robot/Kinematics/Forward Kinematics/Simulink Function ==
  Transform : TriggerPort  TriggerType=function-call  IsSimulinkFunction=on  FunctionName=Transform  FunctionVisibility=scoped  VariantControl=(inherit)
  MATLAB Function : MATLAB Function  TreatAsAtomicUnit=on
  q : ArgIn  DisableCoverage=on  PortDimensions=[1 20]  ArgumentName=q
  Thead : ArgOut  DisableCoverage=on  PortDimensions=[4 4]  ArgumentName=Thead
  Trleg : ArgOut  DisableCoverage=on  Port=2  PortDimensions=[4 4]  ArgumentName=Trleg
  Tlleg : ArgOut  DisableCoverage=on  Port=3  PortDimensions=[4 4]  ArgumentName=Tlleg
  Trarm : ArgOut  Port=4  PortDimensions=[4 4]  ArgumentName=Trarm
  Tlarm : ArgOut  Port=5  PortDimensions=[4 4]  ArgumentName=Tlarm
  wires:
  q/1 -> MATLAB Function/1(q)
  MATLAB Function/1(Thead) -> Thead/1
  MATLAB Function/3(Tlleg) -> Tlleg/1
  MATLAB Function/2(Trleg) -> Trleg/1
  MATLAB Function/4(Trarm) -> Trarm/1
  MATLAB Function/5(Tlarm) -> Tlarm/1

== system Robot/Kinematics/Invesre Kinematics/Simulink Function ==
  InverseTransform : TriggerPort  TriggerType=function-call  IsSimulinkFunction=on  FunctionName=InverseTransform  FunctionVisibility=scoped  VariantControl=(inherit)
  MATLAB Function : MATLAB Function  TreatAsAtomicUnit=on
  xhead : ArgIn  DisableCoverage=on  ArgumentName=xhead
  yhead : ArgIn  Port=2  ArgumentName=yhead
  zhead : ArgIn  Port=3  ArgumentName=zhead
  pLLeg : ArgIn  Port=4  PortDimensions=[1 6]  ArgumentName=pLLeg
  pRLeg : ArgIn  Port=5  PortDimensions=[1 6]  ArgumentName=pRLeg
  pTorso : ArgIn  Port=6  PortDimensions=[1 6]  ArgumentName=pTorso
  legSupport : ArgIn  Port=7  ArgumentName=legSupport
  transLArm : ArgIn  Port=8  PortDimensions=[4 4]  ArgumentName=transLArm
  transRArm : ArgIn  Port=9  PortDimensions=[4 4]  ArgumentName=transRArm
  q1 : ArgOut  DisableCoverage=on  ArgumentName=q1
  q2 : ArgOut  DisableCoverage=on  Port=2  ArgumentName=q2
  q3 : ArgOut  DisableCoverage=on  Port=3  ArgumentName=q3
  q4 : ArgOut  Port=4  ArgumentName=q4
  qLegs : ArgOut  Port=5  PortDimensions=[1 12]  ArgumentName=qLegs
  qLArms : ArgOut  Port=6  PortDimensions=[1 5]  ArgumentName=qLArms
  qRArms : ArgOut  Port=7  PortDimensions=[1 5]  ArgumentName=qRArms
  wires:
  xhead/1 -> MATLAB Function/1(xhead)
  MATLAB Function/1(q1) -> q1/1
  MATLAB Function/2(q2) -> q2/1
  MATLAB Function/3(q3) -> q3/1
  zhead/1 -> MATLAB Function/3(zhead)
  yhead/1 -> MATLAB Function/2(yhead)
  MATLAB Function/4(q4) -> q4/1
  pLLeg/1 -> MATLAB Function/4(pLLeg)
  pRLeg/1 -> MATLAB Function/5(pRLeg)
  pTorso/1 -> MATLAB Function/6(pTorso)
  legSupport/1 -> MATLAB Function/7(legSupport)
  MATLAB Function/5(qLegs) -> qLegs/1
  MATLAB Function/6(qLArms) -> qLArms/1
  MATLAB Function/7(qRArms) -> qRArms/1
  transLArm/1 -> MATLAB Function/8(transLArm)
  transRArm/1 -> MATLAB Function/9(transRArm)

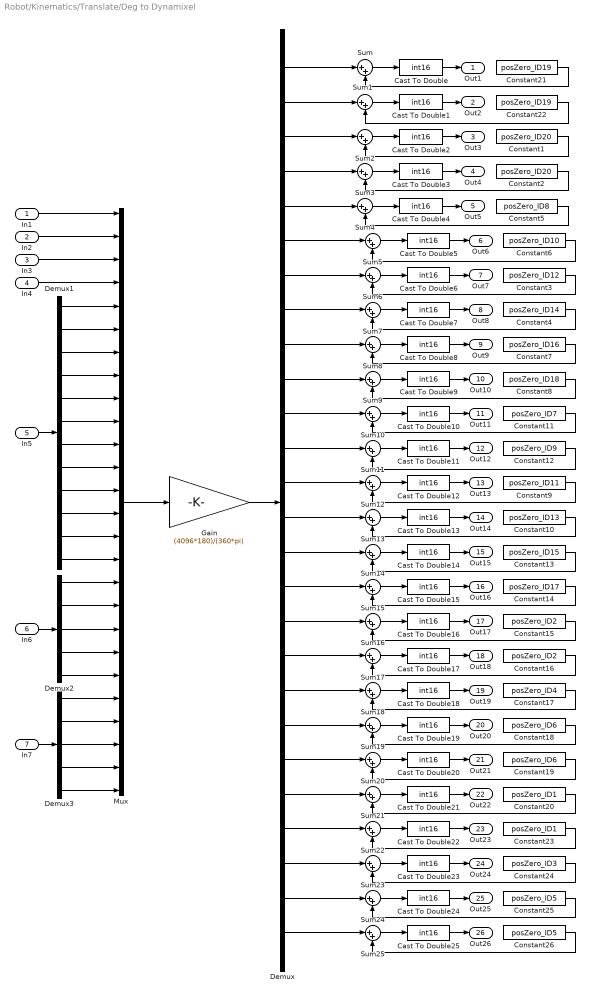
== system Robot/Kinematics/Translate/Deg to Dynamixel ==
  In1 : Inport
  In2 : Inport  Port=2
  In3 : Inport  Port=3
  In4 : Inport  Port=4
  In5 : Inport  Port=5
  In6 : Inport  Port=6
  In7 : Inport  Port=7
  Cast To Double{,1..25} (26 alike) : DataTypeConversion  OutDataTypeStr=int16
  Constant1 : Constant  Value=posZero_ID20  OutDataTypeStr=int16
  Constant10 : Constant  Value=posZero_ID13  OutDataTypeStr=int16
  Constant11 : Constant  Value=posZero_ID7  OutDataTypeStr=int16
  Constant12 : Constant  Value=posZero_ID9  OutDataTypeStr=int16
  Constant13 : Constant  Value=posZero_ID15  OutDataTypeStr=int16
  Constant14 : Constant  Value=posZero_ID17  OutDataTypeStr=int16
  Constant15 : Constant  Value=posZero_ID2  OutDataTypeStr=int16
  Constant16 : Constant  Value=posZero_ID2  OutDataTypeStr=int16
  Constant17 : Constant  Value=posZero_ID4  OutDataTypeStr=int16
  Constant18 : Constant  Value=posZero_ID6  OutDataTypeStr=int16
  Constant19 : Constant  Value=posZero_ID6  OutDataTypeStr=int16
  Constant2 : Constant  Value=posZero_ID20  OutDataTypeStr=int16
  Constant20 : Constant  Value=posZero_ID1  OutDataTypeStr=int16
  Constant21 : Constant  Value=posZero_ID19  OutDataTypeStr=int16
  Constant22 : Constant  Value=posZero_ID19  OutDataTypeStr=int16
  Constant23 : Constant  Value=posZero_ID1  OutDataTypeStr=int16
  Constant24 : Constant  Value=posZero_ID3  OutDataTypeStr=int16
  Constant25 : Constant  Value=posZero_ID5  OutDataTypeStr=int16
  Constant26 : Constant  Value=posZero_ID5  OutDataTypeStr=int16
  Constant3 : Constant  Value=posZero_ID12  OutDataTypeStr=int16
  Constant4 : Constant  Value=posZero_ID14  OutDataTypeStr=int16
  Constant5 : Constant  Value=posZero_ID8  OutDataTypeStr=int16
  Constant6 : Constant  Value=posZero_ID10  OutDataTypeStr=int16
  Constant7 : Constant  Value=posZero_ID16  OutDataTypeStr=int16
  Constant8 : Constant  Value=posZero_ID18  OutDataTypeStr=int16
  Constant9 : Constant  Value=posZero_ID11  OutDataTypeStr=int16
  Demux : Demux  Outputs=26
  Demux1 : Demux  Outputs=12
  Demux2 : Demux  Outputs=5
  Demux3 : Demux  Outputs=5
  Gain : Gain  Gain=(4096*180)/(360*pi)  SaturateOnIntegerOverflow=on  OutDataTypeStr=Inherit: Same as input
  Mux : Mux  Inputs=26
  Sum{,1..25} (26 alike) : Sum  Inputs=|++
  Out1 : Outport
  Out2 : Outport  Port=2
  Out3 : Outport  Port=3
  Out4 : Outport  Port=4
  Out5 : Outport  Port=5
  Out6 : Outport  Port=6
  Out7 : Outport  Port=7
  Out8 : Outport  Port=8
  Out9 : Outport  Port=9
  Out10 : Outport  Port=10
  Out11 : Outport  Port=11
  Out12 : Outport  Port=12
  Out13 : Outport  Port=13
  Out14 : Outport  Port=14
  Out15 : Outport  Port=15
  Out16 : Outport  Port=16
  Out17 : Outport  Port=17
  Out18 : Outport  Port=18
  Out19 : Outport  Port=19
  Out20 : Outport  Port=20
  Out21 : Outport  Port=21
  Out22 : Outport  Port=22
  Out23 : Outport  Port=23
  Out24 : Outport  Port=24
  Out25 : Outport  Port=25
  Out26 : Outport  Port=26
  wires:
  Demux/3 -> Sum2/1
  Constant1/1 -> Sum2/2
  Sum2/1 -> Cast To Double2/1
  Constant22/1 -> Sum1/2
  Demux/2 -> Sum1/1
  Sum/1 -> Cast To Double/1
  Constant21/1 -> Sum/2
  Demux/1 -> Sum/1
  Gain/1 -> Demux/1
  Mux/1 -> Gain/1
  Sum3/1 -> Cast To Double3/1
  Constant2/1 -> Sum3/2
  Demux/4 -> Sum3/1
  Cast To Double/1 -> Out1/1
  Sum1/1 -> Cast To Double1/1
  Cast To Double1/1 -> Out2/1
  Cast To Double2/1 -> Out3/1
  Cast To Double3/1 -> Out4/1
  In5/1 -> Demux1/1
  Cast To Double7/1 -> Out8/1
  Cast To Double6/1 -> Out7/1
  Cast To Double5/1 -> Out6/1
  Sum5/1 -> Cast To Double5/1
  Cast To Double4/1 -> Out5/1
  Demux/8 -> Sum7/1
  Constant4/1 -> Sum7/2
  Sum7/1 -> Cast To Double7/1
  Demux/5 -> Sum4/1
  Constant5/1 -> Sum4/2
  Sum4/1 -> Cast To Double4/1
  Demux/6 -> Sum5/1
  Constant6/1 -> Sum5/2
  Sum6/1 -> Cast To Double6/1
  Constant3/1 -> Sum6/2
  Demux/7 -> Sum6/1
  Demux/9 -> Sum8/1
  Constant7/1 -> Sum8/2
  Sum8/1 -> Cast To Double8/1
  Sum9/1 -> Cast To Double9/1
  Constant8/1 -> Sum9/2
  Demux/10 -> Sum9/1
  Cast To Double8/1 -> Out9/1
  Cast To Double9/1 -> Out10/1
  Cast To Double15/1 -> Out16/1
  Cast To Double14/1 -> Out15/1
  Demux/16 -> Sum15/1
  Constant14/1 -> Sum15/2
  Sum15/1 -> Cast To Double15/1
  Sum14/1 -> Cast To Double14/1
  Constant13/1 -> Sum14/2
  Demux/15 -> Sum14/1
  Demux/13 -> Sum12/1
  Constant9/1 -> Sum12/2
  Sum12/1 -> Cast To Double12/1
  Constant12/1 -> Sum11/2
  Sum10/1 -> Cast To Double10/1
  Constant11/1 -> Sum10/2
  Demux/11 -> Sum10/1
  Sum13/1 -> Cast To Double13/1
  Constant10/1 -> Sum13/2
  Demux/14 -> Sum13/1
  Cast To Double10/1 -> Out11/1
  Sum11/1 -> Cast To Double11/1
  Cast To Double11/1 -> Out12/1
  Cast To Double12/1 -> Out13/1
  Cast To Double13/1 -> Out14/1
  Demux/12 -> Sum11/1
  In6/1 -> Demux2/1
  In7/1 -> Demux3/1
  In1/1 -> Mux/1
  In2/1 -> Mux/2
  In3/1 -> Mux/3
  In4/1 -> Mux/4
  Demux1/1 -> Mux/5
  Demux1/2 -> Mux/6
  Demux1/3 -> Mux/7
  Demux1/4 -> Mux/8
  Demux1/5 -> Mux/9
  Demux1/6 -> Mux/10
  Demux1/7 -> Mux/11
  Demux1/8 -> Mux/12
  Demux1/9 -> Mux/13
  Demux1/10 -> Mux/14
  Demux1/11 -> Mux/15
  Demux1/12 -> Mux/16
  Demux/17 -> Sum16/1
  Constant15/1 -> Sum16/2
  Sum16/1 -> Cast To Double16/1
  Cast To Double16/1 -> Out17/1
  Demux/18 -> Sum17/1
  Constant16/1 -> Sum17/2
  Sum17/1 -> Cast To Double17/1
  Cast To Double17/1 -> Out18/1
  Demux/19 -> Sum18/1
  Constant17/1 -> Sum18/2
  Sum18/1 -> Cast To Double18/1
  Cast To Double18/1 -> Out19/1
  Demux/20 -> Sum19/1
  Constant18/1 -> Sum19/2
  Sum19/1 -> Cast To Double19/1
  Cast To Double19/1 -> Out20/1
  Demux/21 -> Sum20/1
  Constant19/1 -> Sum20/2
  Sum20/1 -> Cast To Double20/1
  Cast To Double20/1 -> Out21/1
  Demux/22 -> Sum21/1
  Constant20/1 -> Sum21/2
  Sum21/1 -> Cast To Double21/1
  Cast To Double21/1 -> Out22/1
  Demux2/1 -> Mux/17
  Demux2/2 -> Mux/18
  Demux2/3 -> Mux/19
  Demux2/4 -> Mux/20
  Demux2/5 -> Mux/21
  Demux3/1 -> Mux/22
  Demux3/2 -> Mux/23
  Demux3/5 -> Mux/26
  Demux3/3 -> Mux/24
  Demux3/4 -> Mux/25
  Demux/23 -> Sum22/1
  Cast To Double22/1 -> Out23/1
  Sum22/1 -> Cast To Double22/1
  Constant23/1 -> Sum22/2
  Demux/24 -> Sum23/1
  Cast To Double23/1 -> Out24/1
  Sum23/1 -> Cast To Double23/1
  Constant24/1 -> Sum23/2
  Demux/25 -> Sum24/1
  Cast To Double24/1 -> Out25/1
  Sum24/1 -> Cast To Double24/1
  Constant25/1 -> Sum24/2
  Demux/26 -> Sum25/1
  Cast To Double25/1 -> Out26/1
  Sum25/1 -> Cast To Double25/1
  Constant26/1 -> Sum25/2

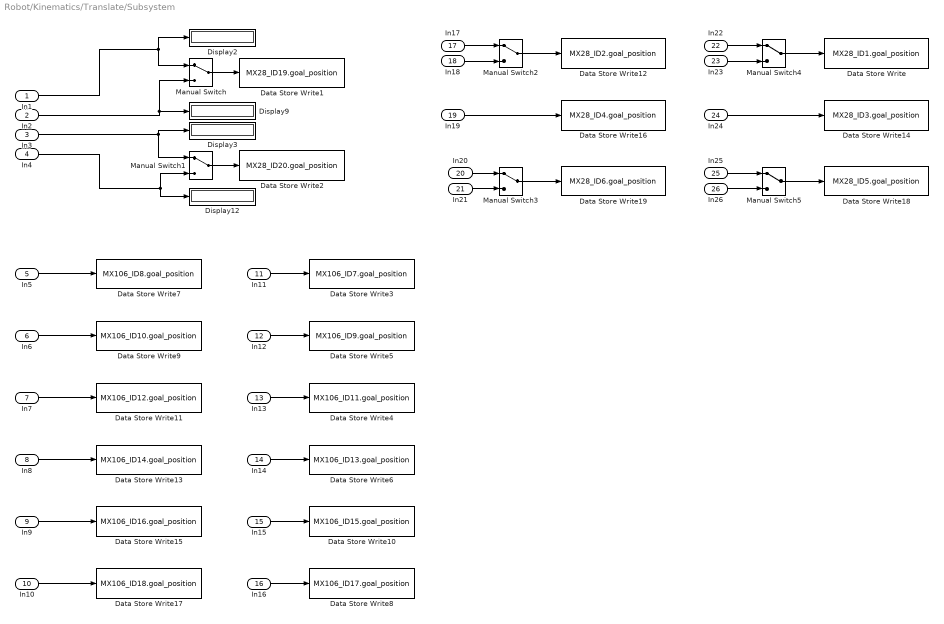
== system Robot/Kinematics/Translate/Subsystem ==
  In1 : Inport
  In2 : Inport  Port=2
  In3 : Inport  Port=3
  In4 : Inport  Port=4
  In5 : Inport  Port=5
  In6 : Inport  Port=6
  In7 : Inport  Port=7
  In8 : Inport  Port=8
  In9 : Inport  Port=9
  In10 : Inport  Port=10
  In11 : Inport  Port=11
  In12 : Inport  Port=12
  In13 : Inport  Port=13
  In14 : Inport  Port=14
  In15 : Inport  Port=15
  In16 : Inport  Port=16
  In17 : Inport  Port=17
  In18 : Inport  Port=18
  In19 : Inport  Port=19
  In20 : Inport  Port=20
  In21 : Inport  Port=21
  In22 : Inport  Port=22
  In23 : Inport  Port=23
  In24 : Inport  Port=24
  In25 : Inport  Port=25
  In26 : Inport  Port=26
  Data Store Write : DataStoreWrite  DataStoreName=MX28_ID1  DataStoreElements=MX28_ID1.goal_position
  Data Store Write1 : DataStoreWrite  DataStoreName=MX28_ID19  DataStoreElements=MX28_ID19.goal_position
  Data Store Write10 : DataStoreWrite  DataStoreName=MX106_ID15  DataStoreElements=MX106_ID15.goal_position
  Data Store Write11 : DataStoreWrite  DataStoreName=MX106_ID12  DataStoreElements=MX106_ID12.goal_position
  Data Store Write12 : DataStoreWrite  DataStoreName=MX28_ID2  DataStoreElements=MX28_ID2.goal_position
  Data Store Write13 : DataStoreWrite  DataStoreName=MX106_ID14  DataStoreElements=MX106_ID14.goal_position
  Data Store Write14 : DataStoreWrite  DataStoreName=MX28_ID3  DataStoreElements=MX28_ID3.goal_position
  Data Store Write15 : DataStoreWrite  DataStoreName=MX106_ID16  DataStoreElements=MX106_ID16.goal_position
  Data Store Write16 : DataStoreWrite  DataStoreName=MX28_ID4  DataStoreElements=MX28_ID4.goal_position
  Data Store Write17 : DataStoreWrite  DataStoreName=MX106_ID18  DataStoreElements=MX106_ID18.goal_position
  Data Store Write18 : DataStoreWrite  DataStoreName=MX28_ID5  DataStoreElements=MX28_ID5.goal_position
  Data Store Write19 : DataStoreWrite  DataStoreName=MX28_ID6  DataStoreElements=MX28_ID6.goal_position
  Data Store Write2 : DataStoreWrite  DataStoreName=MX28_ID20  DataStoreElements=MX28_ID20.goal_position
  Data Store Write3 : DataStoreWrite  DataStoreName=MX106_ID7  DataStoreElements=MX106_ID7.goal_position
  Data Store Write4 : DataStoreWrite  DataStoreName=MX106_ID11  DataStoreElements=MX106_ID11.goal_position
  Data Store Write5 : DataStoreWrite  DataStoreName=MX106_ID9  DataStoreElements=MX106_ID9.goal_position
  Data Store Write6 : DataStoreWrite  DataStoreName=MX106_ID13  DataStoreElements=MX106_ID13.goal_position
  Data Store Write7 : DataStoreWrite  DataStoreName=MX106_ID8  DataStoreElements=MX106_ID8.goal_position
  Data Store Write8 : DataStoreWrite  DataStoreName=MX106_ID17  DataStoreElements=MX106_ID17.goal_position
  Data Store Write9 : DataStoreWrite  DataStoreName=MX106_ID10  DataStoreElements=MX106_ID10.goal_position
  Display{2..3,9,12} (4 alike) : Display
      settings: Format=bank
  Manual Switch{,1..5} (6 alike) : ManualSwitch
  wires:
  Manual Switch1/1 -> Data Store Write2/1
  In2/1 -> Manual Switch/2, Display9/1
  In3/1 -> Manual Switch1/1, Display3/1
  In4/1 -> Display12/1, Manual Switch1/2
  Manual Switch/1 -> Data Store Write1/1
  In1/1 -> Display2/1, Manual Switch/1
  In8/1 -> Data Store Write13/1
  In11/1 -> Data Store Write3/1
  In14/1 -> Data Store Write6/1
  In6/1 -> Data Store Write9/1
  In7/1 -> Data Store Write11/1
  In10/1 -> Data Store Write17/1
  In9/1 -> Data Store Write15/1
  In12/1 -> Data Store Write5/1
  In13/1 -> Data Store Write4/1
  In15/1 -> Data Store Write10/1
  In16/1 -> Data Store Write8/1
  In5/1 -> Data Store Write7/1
  Manual Switch2/1 -> Data Store Write12/1
  In17/1 -> Manual Switch2/1
  In18/1 -> Manual Switch2/2
  In19/1 -> Data Store Write16/1
  In22/1 -> Manual Switch4/1
  In23/1 -> Manual Switch4/2
  Manual Switch4/1 -> Data Store Write/1
  In24/1 -> Data Store Write14/1
  Manual Switch5/1 -> Data Store Write18/1
  In25/1 -> Manual Switch5/1
  In26/1 -> Manual Switch5/2
  In20/1 -> Manual Switch3/1
  In21/1 -> Manual Switch3/2
  Manual Switch3/1 -> Data Store Write19/1

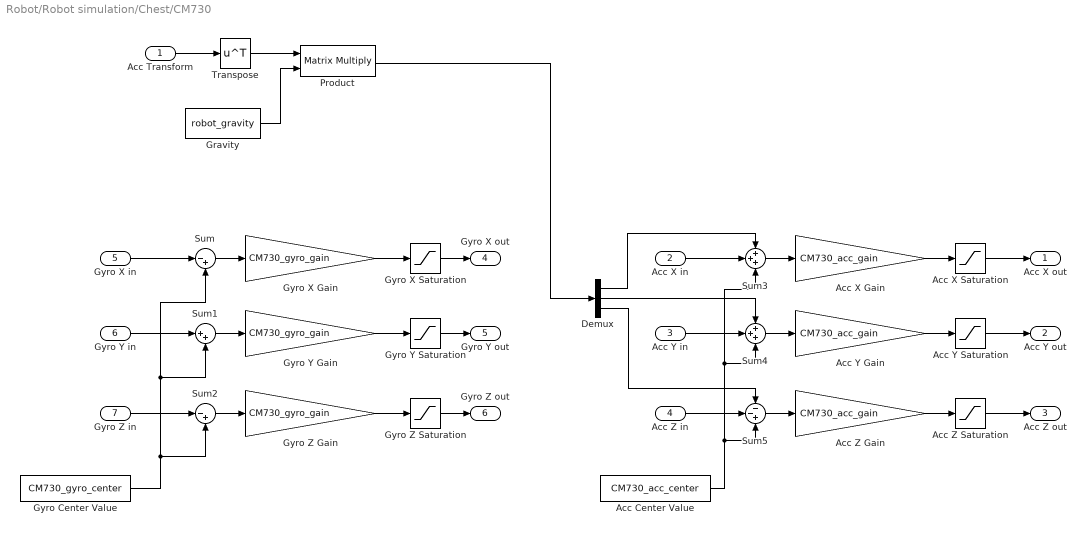
== system Robot/Robot simulation/Chest/CM730 ==
  Acc Transform : Inport
  Acc X in : Inport  Port=2
  Acc Y in : Inport  Port=3
  Acc Z in : Inport  Port=4
  Gyro X in : Inport  Port=5
  Gyro Y in : Inport  Port=6
  Gyro Z in : Inport  Port=7
  Acc Center Value : Constant  Value=CM730_acc_center
  Acc X Gain : Gain  Gain=CM730_acc_gain  OutMax=1023  OutDataTypeStr=int16  SaturateOnIntegerOverflow=on
  Acc X Saturation : Saturate  UpperLimit=1023  LowerLimit=0
  Acc Y Gain : Gain  Gain=CM730_acc_gain  OutDataTypeStr=int16  SaturateOnIntegerOverflow=on
  Acc Y Saturation : Saturate  UpperLimit=1023  LowerLimit=0
  Acc Z Gain : Gain  Gain=CM730_acc_gain  OutDataTypeStr=int16  SaturateOnIntegerOverflow=on
  Acc Z Saturation : Saturate  UpperLimit=1023  LowerLimit=0
  Demux : Demux  Outputs=3
  Gravity : Constant  Value=robot_gravity
  Gyro Center Value : Constant  Value=CM730_gyro_center
  Gyro X Gain : Gain  Gain=CM730_gyro_gain  OutDataTypeStr=int16  SaturateOnIntegerOverflow=on
  Gyro X Saturation : Saturate  UpperLimit=1023  LowerLimit=0
  Gyro Y Gain : Gain  Gain=CM730_gyro_gain  OutDataTypeStr=int16  SaturateOnIntegerOverflow=on
  Gyro Y Saturation : Saturate  UpperLimit=1023  LowerLimit=0
  Gyro Z Gain : Gain  Gain=CM730_gyro_gain  OutDataTypeStr=int16  SaturateOnIntegerOverflow=on
  Gyro Z Saturation : Saturate  UpperLimit=1023  LowerLimit=0
  Product : Product  Multiplication=Matrix(*)
  Sum : Sum  Inputs=|-+
  Sum1 : Sum  Inputs=|++
  Sum2 : Sum  Inputs=|-+
  Sum3 : Sum  Inputs=+++
  Sum4 : Sum  Inputs=+++
  Sum5 : Sum  Inputs=--+
  Transpose : Math  Operator=transpose  SaturateOnIntegerOverflow=on
  Acc X out : Outport
  Acc Y out : Outport  Port=2
  Acc Z out : Outport  Port=3
  Gyro X out : Outport  Port=4
  Gyro Y out : Outport  Port=5
  Gyro Z out : Outport  Port=6
  wires:
  Gyro X Gain/1 -> Gyro X Saturation/1
  Gyro Y Gain/1 -> Gyro Y Saturation/1
  Product/1 -> Demux/1
  Acc X Gain/1 -> Acc X Saturation/1
  Acc Y Gain/1 -> Acc Y Saturation/1
  Acc Z Gain/1 -> Acc Z Saturation/1
  Sum/1 -> Gyro X Gain/1
  Gyro X in/1 -> Sum/1
  Sum2/1 -> Gyro Z Gain/1
  Gyro Z in/1 -> Sum2/1
  Gyro Y in/1 -> Sum1/1
  Sum1/1 -> Gyro Y Gain/1
  Gyro Center Value/1 -> Sum2/2, Sum1/2, Sum/2
  Sum3/1 -> Acc X Gain/1
  Acc X in/1 -> Sum3/2
  Acc Y in/1 -> Sum4/2
  Sum4/1 -> Acc Y Gain/1
  Sum5/1 -> Acc Z Gain/1
  Acc Z in/1 -> Sum5/2
  Acc Center Value/1 -> Sum5/3, Sum4/3, Sum3/3
  Demux/1 -> Sum3/1
  Demux/2 -> Sum4/1
  Demux/3 -> Sum5/1
  Gyro Z Gain/1 -> Gyro Z Saturation/1
  Acc Transform/1 -> Transpose/1
  Gravity/1 -> Product/2
  Transpose/1 -> Product/1
  Gyro X Saturation/1 -> Gyro X out/1
  Gyro Y Saturation/1 -> Gyro Y out/1
  Gyro Z Saturation/1 -> Gyro Z out/1
  Acc X Saturation/1 -> Acc X out/1
  Acc Y Saturation/1 -> Acc Y out/1
  Acc Z Saturation/1 -> Acc Z out/1
